simulink model "sim_part2"  (R2022a)
settings: Solver=VariableStepAuto  StartTime=0.0  StopTime=0.4  RelTol=1e-3
values from neighbouring files (symbols this model uses):
  A = [0 1 0             0 ... (first row only)    [Prep.m]    (also in prelab.m = [0 1 0 0; 0 0 -m*g / M 0; 0 0 0 1; 0 0 (M+m)*g/(M*l) 0])
  A2 = double(subs(A))    [Prep.m]    (also in prelab.m = [0 1 0 0; 0 0 -m*g / M 0; 0 0 0 1; 0 0 (M+m)*g/(M*l) 0])
  A3 = double(subs(A))    [Prep.m]    (also in prelab.m = [0 1 0 0; 0 0 -m*g / M 0; 0 0 0 1; 0 0 (M+m)*g/(M*l) 0])
  B = [0 ... (first row only)    [Prep.m]    (also in prelab.m = [0; 1/M; 0; -1/(M*l)])
  B2 = double(subs(B))    [Prep.m]    (also in prelab.m = [0; 1/M; 0; -1/(M*l)])
  B3 = double(subs(B))    [Prep.m]    (also in prelab.m = [0; 1/M; 0; -1/(M*l)])
  C = eye(4)    [prelab.m]
  C2 = eye(4)    [prelab.m]
  C3 = eye(4)    [prelab.m]
  D = [0;0;0;0]    [prelab.m]
  D2 = [0;0;0;0]    [prelab.m]
  D3 = [0;0;0;0]    [prelab.m]
libraries: truetime x1
settings Model: Creator=lixinru  LastModifiedBy=theod
settings DebuggingCC: UnconnectedInputMsg=warning  UnconnectedOutputMsg=warning  UnconnectedLineMsg=warning
settings RTWCC: DLArmComputeVersion=19.05

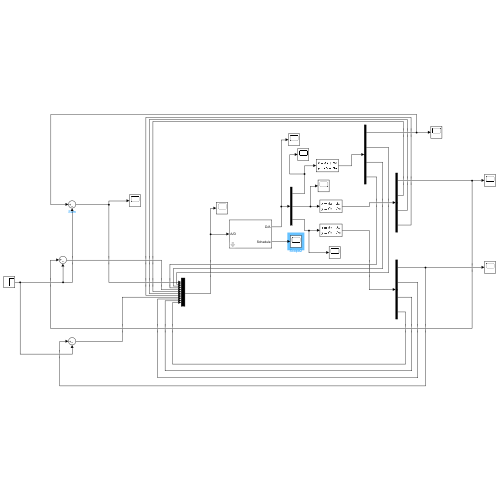
[thumbnail: Simulink's stored preview of the top-level diagram]
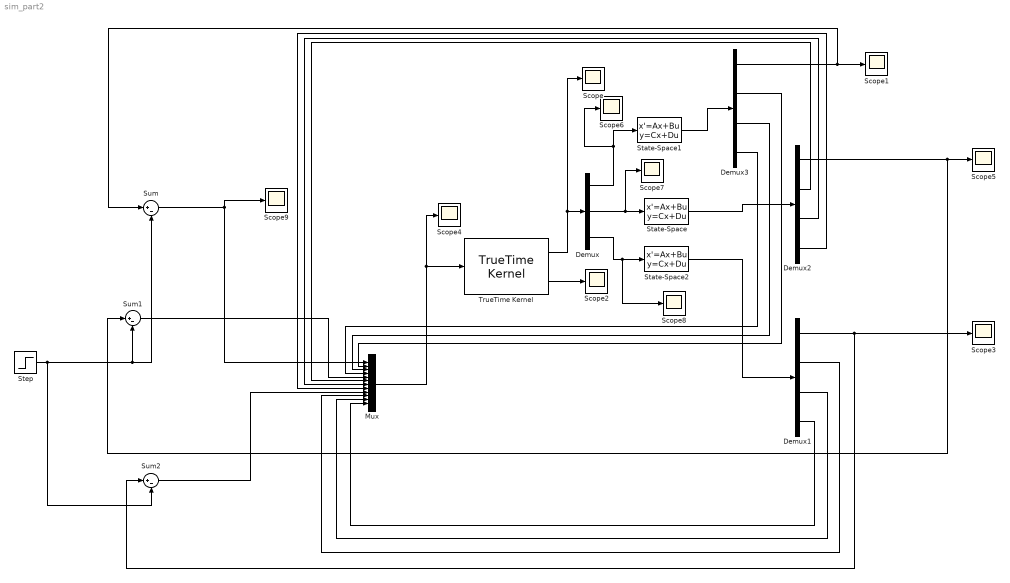
== system sim_part2 ==
  Demux : Demux  Outputs=3
  Demux1 : Demux
      settings: DisplayOption=none
  Demux2 : Demux
      settings: DisplayOption=none
  Demux3 : Demux
      settings: DisplayOption=none
  Mux : Mux  Inputs=12
  Scope{,1..9} (10 alike) : Scope
  State-Space : StateSpace  A=A2  B=B2  C=C2  D=D2  InitialCondition=0
  State-Space1 : StateSpace  A=A  B=B  C=C  D=D  InitialCondition=0  ParameterTunability=Optimized
  State-Space2 : StateSpace  A=A3  B=B3  C=C3  D=D3  InitialCondition=0
  Step : Step  Time=0  Before=1  SampleTime=0
  Sum : Sum  Inputs=|+-
  Sum1 : Sum  Inputs=|+-
  Sum2 : Sum  Inputs=|+-
  TrueTime Kernel : truetime/TrueTime Kernel  sfun=node_init  args=[]  ninputsoutputs=[12 3]  ntriggers=0  trigtype=falling  nwnodenbr=[]  clockoffsetdrift=[0 0]  schedoutput=on  battery=off  poweroutput=off
  wires:
  Mux/1 -> TrueTime Kernel/1, Scope4/1
  Demux/3 -> Scope8/1, State-Space2/1
  TrueTime Kernel/2 -> Scope2/1
  TrueTime Kernel/1 -> Scope/1, Demux/1
  State-Space2/1 -> Demux1/1
  Demux1/1 -> Sum2/1, Scope3/1
  Demux2/1 -> Sum1/1, Scope5/1
  Demux1/4 -> Mux/12
  Demux1/3 -> Mux/11
  Demux1/2 -> Mux/10
  Demux2/4 -> Mux/8
  Demux2/3 -> Mux/7
  Demux2/2 -> Mux/6
  Demux3/4 -> Mux/4
  Demux3/3 -> Mux/3
  Demux3/2 -> Mux/2
  Demux3/1 -> Sum/1, Scope1/1
  Step/1 -> Sum2/2, Sum1/2, Sum/2
  Sum2/1 -> Mux/9
  Sum1/1 -> Mux/5
  Sum/1 -> Mux/1, Scope9/1
  Demux/2 -> Scope7/1, State-Space/1
  State-Space/1 -> Demux2/1
  State-Space1/1 -> Demux3/1
  Demux/1 -> Scope6/1, State-Space1/1
